simulink model "sim8_1"  (R2019a)
settings: Solver=VariableStepAuto  StartTime=0.0  StopTime=10.0  RelTol=1e-3
values from neighbouring files (symbols this model uses):
  C = [1 0]    [matlab8_1.m]
  C2 = [0 1]    [matlab8_1.m]
  Csim = eye(2)    [matlab8_1.m]
  Dsim = [0; 0]    [matlab8_1.m]
  gamma = [2; 1]    [matlab8_1.m]
  h = wnh / wn    [matlab8_1.m]
  L = [0  1] * inv(Wc) * (phi^2 + p1 * phi + p2 * eye(2))    [matlab8_1.m]
  Lc = G_dc / (C * inv(eye(2) - phi_cl) * gamma)    [matlab8_1.m]
  phi = [1 phi_12; 0 0.4]    [matlab8_1.m]
settings Model: Creator=User  LastModifiedBy=User

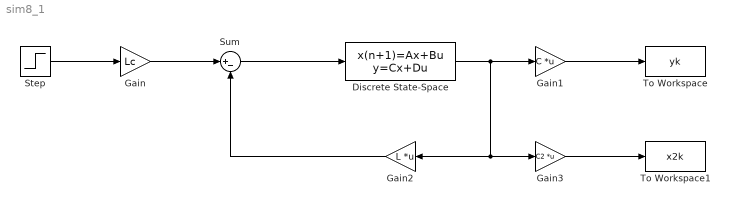
== system sim8_1 ==
  Discrete State-Space : DiscreteStateSpace  A=phi  B=gamma  C=Csim  D=Dsim  SampleTime=h
  Gain : Gain  Gain=Lc
  Gain1 : Gain  Gain=C  Multiplication=Matrix(K*u) (u vector)
  Gain2 : Gain  Gain=L  Multiplication=Matrix(K*u) (u vector)
  Gain3 : Gain  Gain=C2  Multiplication=Matrix(K*u) (u vector)
  Step : Step  SampleTime=0
  Sum : Sum  Inputs=|+-
  To Workspace : ToWorkspace  VariableName=yk  SaveFormat=Structure With Time  SampleTime=-1
  To Workspace1 : ToWorkspace  VariableName=x2k  SaveFormat=Structure With Time  SampleTime=-1
  wires:
  Step/1 -> Gain/1
  Gain/1 -> Sum/1
  Sum/1 -> Discrete State-Space/1
  Discrete State-Space/1 -> Gain3/1, Gain2/1, Gain1/1
  Gain1/1 -> To Workspace/1
  Gain2/1 -> Sum/2
  Gain3/1 -> To Workspace1/1
